simulink model "Helicopter_DT_sol"  (R2023b)
settings: Solver=ode3  StartTime=0.0  StopTime=10  FixedStep=0.01  RelTol=1e-3
values from neighbouring files (symbols this model uses):
  A = [ -0.4 ,   0 , -0.01 ... (first row only)    [Helicopter_DT_par_sol.m]    (also in Helicopter_par_sol.m)
  B = [ 6.3 ; 0 ; 9.8 ]    [Helicopter_DT_par_sol.m]    (also in Helicopter_par_sol.m)
  C = [ 0 , 0 , 1 ]    [Helicopter_DT_par_sol.m]    (also in Helicopter_par_sol.m)
  K = lqi(sys_DT,Q,R)    [Helicopter_DT_par_sol.m]    (also in Helicopter_par_sol.m = lqr(A,B,Q,R))
  Ts = 0.01    [Helicopter_DT_par_sol.m]    (also in Helicopter_par_sol.m)
settings Model: Creator=jerome  LastModifiedBy=jerome
settings ModelReferenceCC: EnableRefExpFcnMdlSchedulingChecks=on

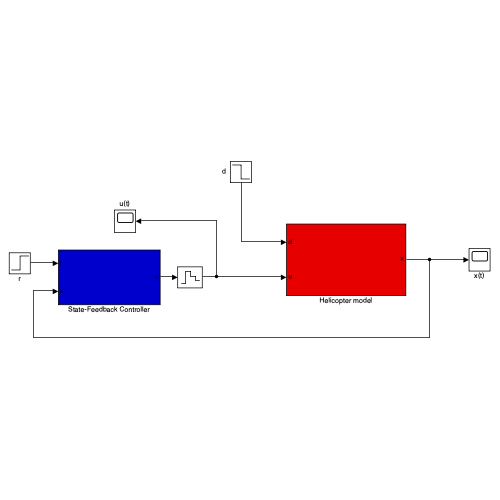
[thumbnail: Simulink's stored preview of the top-level diagram]
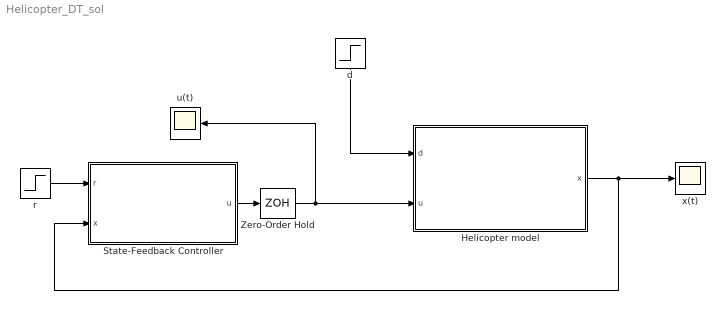
== system Helicopter_DT_sol ==
  Helicopter model : Subsystem
  State-Feedback Controller : Subsystem
  Zero-Order Hold : ZeroOrderHold  SampleTime=Ts
  d : Step  Time=6  After=-1  SampleTime=0
  r : Step  After=10  SampleTime=0
  u(t) : Scope
  x(t) : Scope
  wires:
  Helicopter model/1(x) -> State-Feedback Controller/2(x), x(t)/1
  State-Feedback Controller/1(u) -> Zero-Order Hold/1
  r/1 -> State-Feedback Controller/1(r)
  d/1 -> Helicopter model/1(d)
  Zero-Order Hold/1 -> u(t)/1, Helicopter model/2(u)

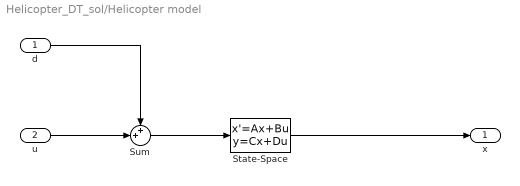
== system Helicopter_DT_sol/Helicopter model ==
  d : Inport
  u : Inport  Port=2
  State-Space : StateSpace  A=A  B=B  C=eye(3)  D=zeros(3,1)  InitialCondition=[0;0;0]
  Sum : Sum  Inputs=++|
  x : Outport
  wires:
  State-Space/1 -> x/1
  Sum/1 -> State-Space/1
  u/1 -> Sum/2
  d/1 -> Sum/1

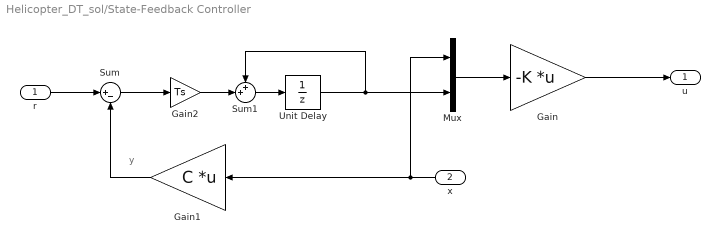
== system Helicopter_DT_sol/State-Feedback Controller ==
  note: y
  r : Inport
  x : Inport  Port=2
  Gain : Gain  Gain=-K  Multiplication=Matrix(K*u) (u vector)
  Gain1 : Gain  Gain=C  Multiplication=Matrix(K*u) (u vector)
  Gain2 : Gain  Gain=Ts
  Mux : Mux  Inputs=2
  Sum : Sum  Inputs=|+-
  Sum1 : Sum  Inputs=++|
  Unit Delay : UnitDelay  SampleTime=-1  HasFrameUpgradeWarning=on
  u : Outport
  wires:
  Gain/1 -> u/1
  Mux/1 -> Gain/1
  r/1 -> Sum/1
  x/1 -> Mux/1, Gain1/1
  Gain1/1 -> Sum/2
  Unit Delay/1 -> Sum1/1, Mux/2
  Sum/1 -> Gain2/1
  Gain2/1 -> Sum1/2
  Sum1/1 -> Unit Delay/1
